simulink model "ParallelForceControl"  (R2020b)
settings: Solver=VariableStepAuto  StartTime=0.0  StopTime=8  RelTol=1e-3
values from neighbouring files (symbols this model uses):
  Fd = [0.1 0 0 0 0 0]    [params.m]
  inv_Md = inv(Md)    [params.m]
  Kd = diag([80 120 50 1 1 1])    [params.m]
  Kf = diag([8 1 1.4 1 1 1])    [params.m]
  Ki = diag([3 1 1.4 1 1 1])    [params.m]
  Kp = diag([200 800 500 1 1 1])    [params.m]
  Md = diag([0.1 1 1 1 1 1])    [params.m]
  xd = Kinematics([t1 d2 d3], param)    [params.m]
libraries: vrlib x1
settings Model: Creator=andre  LastModifiedBy=filippo

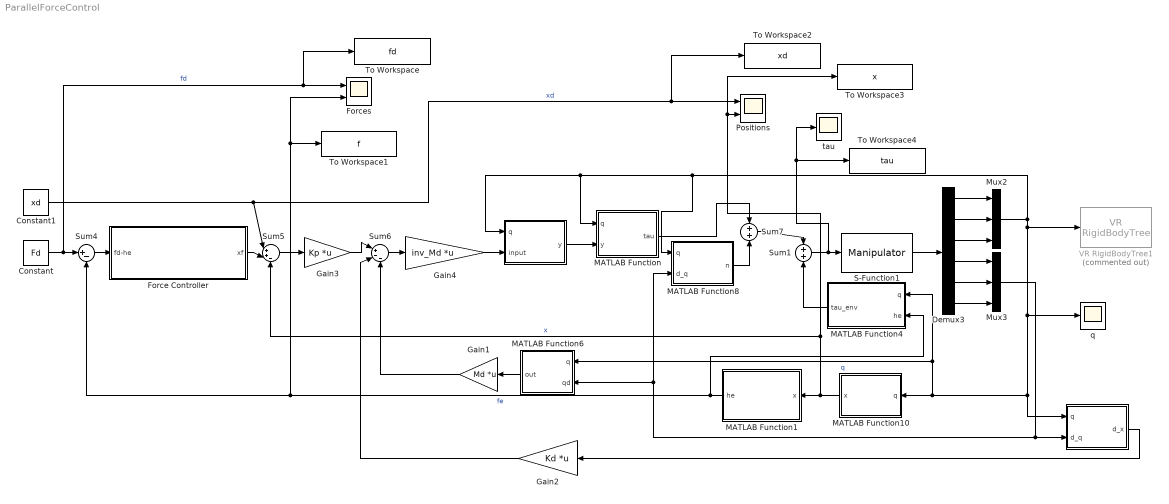
== system ParallelForceControl ==
  " " : MATLAB Function  TreatAsAtomicUnit=on
  "  " : MATLAB Function  TreatAsAtomicUnit=on
  Constant : Constant  Value=Fd
  Constant1 : Constant  Value=xd
  Demux3 : Demux  Outputs=6
  Force Controller : Subsystem
  Forces : Scope  NumInputPorts=2
  Gain1 : Gain  Gain=Md  Multiplication=Matrix(K*u)
  Gain2 : Gain  Gain=Kd  Multiplication=Matrix(K*u)
  Gain3 : Gain  Gain=Kp  Multiplication=Matrix(K*u)
  Gain4 : Gain  Gain=inv_Md  Multiplication=Matrix(K*u)
  MATLAB Function : MATLAB Function  TreatAsAtomicUnit=on
  MATLAB Function1 : MATLAB Function  TreatAsAtomicUnit=on
  MATLAB Function10 : MATLAB Function  TreatAsAtomicUnit=on
  MATLAB Function4 : MATLAB Function  TreatAsAtomicUnit=on
  MATLAB Function6 : MATLAB Function  TreatAsAtomicUnit=on
  MATLAB Function8 : MATLAB Function  TreatAsAtomicUnit=on
  Mux2 : Mux  Inputs=3
  Mux3 : Mux  Inputs=3
  Positions : Scope  NumInputPorts=2
  S-Function1 : S-Function  FunctionName=Manipulator  Parameters=param  SFunctionDeploymentMode=off  EnableBusSupport=off
  Sum1 : Sum
  Sum4 : Sum  Inputs=|+-
  Sum5 : Sum  Inputs=|++-
  Sum6 : Sum  Inputs=|+--
  Sum7 : Sum
  To Workspace : ToWorkspace  VariableName=fd  SaveFormat=Timeseries  SampleTime=-1
  To Workspace1 : ToWorkspace  VariableName=f  SaveFormat=Timeseries  SampleTime=-1
  To Workspace2 : ToWorkspace  VariableName=xd  SaveFormat=Timeseries  SampleTime=-1
  To Workspace3 : ToWorkspace  VariableName=x  SaveFormat=Timeseries  SampleTime=-1
  To Workspace4 : ToWorkspace  VariableName=tau  SaveFormat=Timeseries  SampleTime=-1
  VR RigidBodyTree1 : vrlib/VR RigidBodyTree  Commented=on  RBT=robot  useRBT=on  Ts=-1  ForceViewerOpen=on
      settings: SourceProductBaseCode=SL
  q : Scope
  tau : Scope
  wires:
  Sum4/1 -> Force Controller/1(fd-he)
  Gain4/1 -> " "/2(input)
  Sum6/1 -> Gain4/1
  Sum5/1 -> Gain3/1
  Gain2/1 -> Sum6/2
  Gain3/1 -> Sum6/1
  " "/1(y) -> MATLAB Function/2(y)
  Constant/1 -> To Workspace/1, Forces/1, Sum4/1  "fd"
  MATLAB Function8/1(n) -> Sum7/2
  MATLAB Function/1(tau) -> Sum7/1
  Sum7/1 -> Sum1/1
  Demux3/2 -> Mux2/2
  Demux3/5 -> Mux3/2
  Demux3/3 -> Mux2/3
  Demux3/1 -> Mux2/1
  MATLAB Function1/1(he) -> To Workspace1/1, Forces/2, Sum4/2, MATLAB Function4/2(he)  "fe"
  Demux3/6 -> Mux3/3
  Demux3/4 -> Mux3/1
  S-Function1/1 -> Demux3/1
  MATLAB Function10/1(x) -> Sum5/3, To Workspace3/1, Positions/2, MATLAB Function1/1(x)  "x"
  Mux3/1 -> MATLAB Function6/2(qd), MATLAB Function8/2(d_q), "  "/2(d_q)
  Mux2/1 -> MATLAB Function8/1(q), MATLAB Function/1(q), " "/1(q), VR RigidBodyTree1/1, q/1, "  "/1(q), MATLAB Function4/1(q), MATLAB Function6/1(q), MATLAB Function10/1(q)  "q"
  "  "/1(d_x) -> Gain2/1
  MATLAB Function4/1(tau_env) -> Sum1/2
  Sum1/1 -> To Workspace4/1, tau/1, S-Function1/1
  MATLAB Function6/1(out) -> Gain1/1
  Gain1/1 -> Sum6/3
  Force Controller/1(xf) -> Sum5/2
  Constant1/1 -> Sum5/1, To Workspace2/1, Positions/1  "xd"

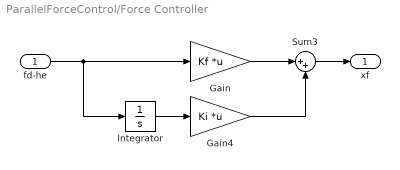
== system ParallelForceControl/Force Controller ==
  fd-he : Inport
  Gain : Gain  Gain=Kf  Multiplication=Matrix(K*u)
  Gain4 : Gain  Gain=Ki  Multiplication=Matrix(K*u)
  Integrator : Integrator
  Sum3 : Sum  Inputs=|++
  xf : Outport
  wires:
  Integrator/1 -> Gain4/1
  Gain/1 -> Sum3/1
  fd-he/1 -> Gain/1, Integrator/1
  Gain4/1 -> Sum3/2
  Sum3/1 -> xf/1

== matlab function ParallelForceControl/MATLAB Function4 ==
  data: q input; he input; tau_env output; param parameter
function tau_env = JT(q, he, param)
    tau_env = -Jacobian(q, param)' * he;
end

== matlab function ParallelForceControl/MATLAB Function6 ==
  data: q input; qd input; out output; param parameter
function out = dot_Ja(q, qd, param)
    d_Ja = AnalyticalJacobian_dot(q,qd,param);
    out = d_Ja * qd;
end

== matlab function ParallelForceControl/MATLAB Function ==
  data: q input; y input; tau output; param parameter
function tau = B(q,y,param)
    B_matrix = B_Lagrangian(q, param);
    tau =  B_matrix * y;
end

== matlab function ParallelForceControl/MATLAB Function8 ==
  data: q input; n output; d_q input; param parameter
function n = n(q,d_q,param)
    % Compute C and G used in the model of n(q,d_q)
    C = double(C_Lagrangian(q, d_q, param));
    G = double(G_Lagrangian(q, param));
    Fsv = param.Fsv;

    n = C * d_q + G + Fsv * d_q;
end

== matlab function ParallelForceControl/   ==
  data: q input; d_x output; d_q input; param parameter
function d_x = Ja(q, d_q, param)
    Ja = AnalyticalJacobian(q,param);
    d_x = Ja * d_q;
end

== matlab function ParallelForceControl/  ==
  data: q input; y output; input input; param parameter
function y = invJa(q, input, param)
    Ja = AnalyticalJacobian(q,param);
    y = pinv(Ja) * input;
end

== matlab function ParallelForceControl/MATLAB Function10 ==
  data: q input; x output; param parameter
function x = Kin(q,param)
    x = Kinematics(q,param);
end

== matlab function ParallelForceControl/MATLAB Function1 ==
  data: x input; he output; param parameter
function he = environment(x, param)
    if x(param.axis) >= param.wall 

        % set up the rest position frame
        xr = zeros(6,1);
        xr(param.axis) = param.wall;

        xe = zeros(6,1);
        xe(param.axis) = x(param.axis);

        he = param.K * (xe - xr);
%         dx_rd = zeros(6,1);
%         dx_rd(2) = xd(2) - xr(2);
%         % At the limit
%         he =  K/(eye(6) + K / KP) * dx_rd;
    else
        he = zeros(6,1);
    end
end
